simulink model "stabilisation_model_lqr"  (R2024b)
settings: Solver=ode3  StartTime=0.0  StopTime=10  FixedStep=1/30  RelTol=1e-3  EnableMultiTasking=on
undefined symbols (not defined in the file): C, D, K, valeurs_calculees
settings Model: Creator=msegui  LastModifiedBy=leofo
settings SolverCC: AlgebraicLoopSolver=TrustRegion
settings DataIOCC: LimitDataPoints=on  SaveFormat=Array  ReturnWorkspaceOutputs=off
settings OptimizationCC: DefaultParameterBehavior=Inlined  BufferReuse=off  ReuseModelBlockBuffer=off  LifeSpan=inf
settings DebuggingCC: UnderspecifiedInitializationDetection=Classic  MergeDetectMultiDrivingBlocksExec=none  SolverPrmCheckMsg=warning  UnconnectedInputMsg=warning  UnconnectedOutputMsg=warning  UnconnectedLineMsg=warning  InitInArrayFormatMsg=none  SFUnexpectedBacktrackingDiag=warning  SFNoUnconditionalDefaultTransitionDiag=warning  ArithmeticOperatorsInVariantConditions=warning
settings HardwareCC: ProdBitPerPointer=32  ProdBitPerSizeT=32  ProdBitPerPtrDiffT=32  ProdLargestAtomicFloat=None  ProdIntDivRoundTo=Undefined  ProdEndianess=Unspecified  ProdWordSize=32  ProdHWDeviceType=32-bit Generic
settings ModelReferenceCC: EnableRefExpFcnMdlSchedulingChecks=on  PropagateSignalLabelsOutOfModel=off
settings SFSimCC: SimUseLocalCustomCode=off  CustomCodeUndefinedFunction=UseInterfaceOnly
settings RTWCC: RTWUseLocalCustomCode=off  GPUComputeCapability=3.5
settings CodeAppCC: StateflowObjectComments=on
settings GRTTargetCC: TargetLangStandard=C89/C90 (ANSI)
settings ConfigComp: CovMetricSettings=dw  CovSaveCumulativeToWorkspaceVar=on  CovSaveSingleToWorkspaceVar=on  CovExternalEMLEnable=off

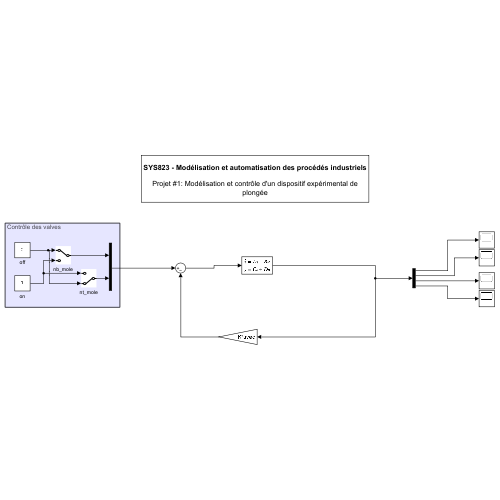
[thumbnail: Simulink's stored preview of the top-level diagram]
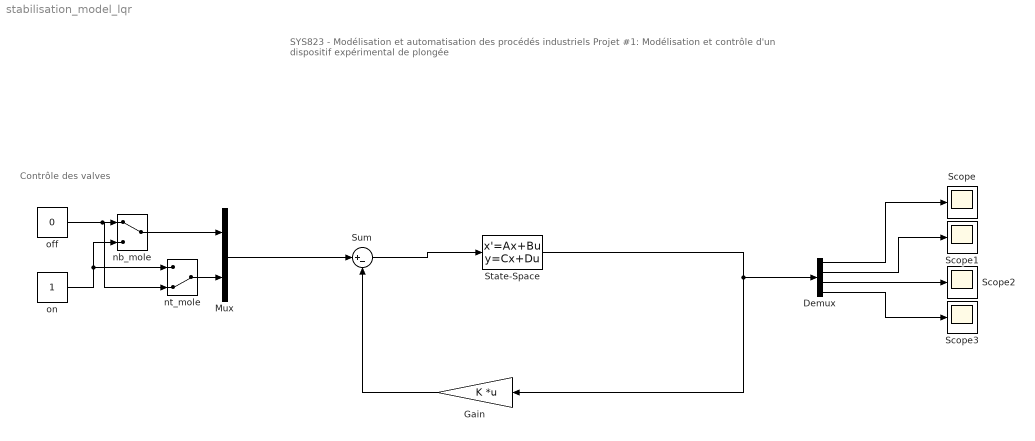
== system stabilisation_model_lqr ==
  note: SYS823 - Modélisation et automatisation des procédés industriels
      |
      | Projet #1: Modélisation et contrôle d'un dispositif expérimental de plongée
  note: Contrôle des valves
  Demux : Demux
  Gain : Gain  Gain=K  Multiplication=Matrix(K*u) (u vector)
  Mux : Mux  Inputs=2
  Scope{,1..3} (4 alike) : Scope
  State-Space : StateSpace  A=valeurs_calculees.A  B=valeurs_calculees.B  C=C  D=D  InitialCondition=[-2.2, 0, valeurs_calculees.n_bonbonne_2m, valeurs_calculees.n_tubes_2m]
  Sum : Sum  Inputs=|+-
  nb_mole : ManualSwitch
  nt_mole : ManualSwitch  CurrentSetting=0
  off : Constant  Value=0
  on : Constant
  wires:
  nb_mole/1 -> Mux/1
  nt_mole/1 -> Mux/2
  off/1 -> nt_mole/2, nb_mole/1
  Demux/1 -> Scope/1
  on/1 -> nt_mole/1, nb_mole/2
  Sum/1 -> State-Space/1
  Mux/1 -> Sum/1
  Demux/2 -> Scope1/1
  Demux/3 -> Scope2/1
  Demux/4 -> Scope3/1
  State-Space/1 -> Gain/1, Demux/1
  Gain/1 -> Sum/2
